simulink model "Testing"  (R2025b)
settings: Solver=VariableStepAuto  StartTime=0.0  StopTime=10.0  RelTol=1e-3
settings Model: Creator=jwjar  LastModifiedBy=jwjar

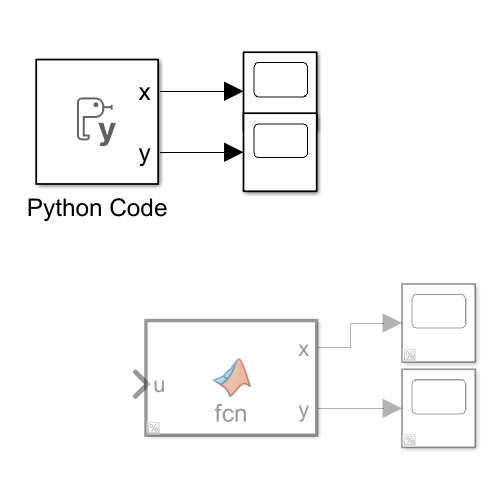
[thumbnail: Simulink's stored preview of the top-level diagram]
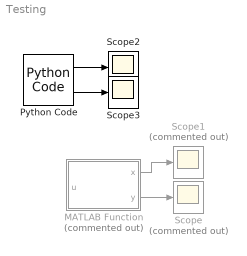
== system Testing ==
  MATLAB Function : MATLAB Function  Commented=on  TreatAsAtomicUnit=on
  Python Code : PythonCode  OutputCode=|
      | import integration.py as functions
      | output = functions.testing()
      | x = output[0]
      | y = output[1]
  Scope : Scope  Commented=on
      settings: ActiveDisplayYMinimum=1  ActiveDisplayYMaximum=3
  Scope1 : Scope  Commented=on
      settings: ActiveDisplayYMinimum=0.9  ActiveDisplayYMaximum=1.1
  Scope2 : Scope
      settings: ActiveDisplayYMinimum=0.9  ActiveDisplayYMaximum=1.1  DataLoggingVariableName=ScopeData2
  Scope3 : Scope
      settings: ActiveDisplayYMinimum=0.9  ActiveDisplayYMaximum=1.1  DataLoggingVariableName=ScopeData3
  wires:
  MATLAB Function/2(y) -> Scope/1
  MATLAB Function/1(x) -> Scope1/1
  Python Code/2 -> Scope3/1
  Python Code/1 -> Scope2/1

== matlab function Testing/MATLAB Function ==
  data: x output; u input; y output
function [x, y]= fcn(u)
x = 0.0;
y = 0.0;
coder.extrinsic("py.integration.testing")
position = py.integration.testing();
x = position(1);
y = position(2);
fprintf("x: %f, y: %f\n", x, y)
end
